simulink model "smd_openloop"  (R2026a)
settings: Solver=VariableStepAuto  StopTime=20
undefined symbols (not defined in the file): c, k, m
settings Model: Creator=tdxt  LastModifiedBy=tdxt

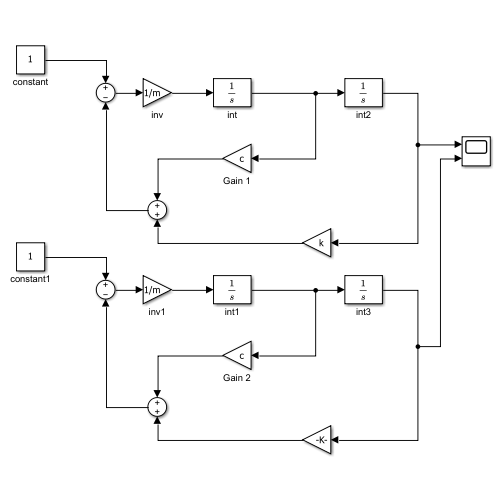
[thumbnail: Simulink's stored preview of the top-level diagram]
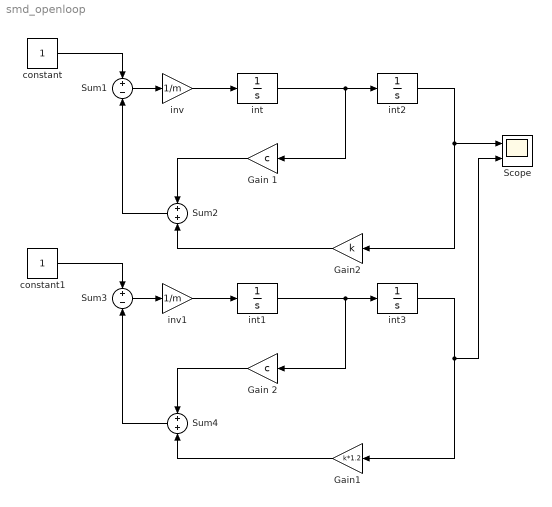
== system smd_openloop ==
  Gain 1 : Gain  Gain=c
  Gain 2 : Gain  Gain=c
  Gain1 : Gain  Gain=k*1.2
  Gain2 : Gain  Gain=k
  Scope : Scope  NumInputPorts=2
      settings: ActiveDisplayYMinimum=-0.14532946588879053  ActiveDisplayYMaximum=1.307965192999115
  Sum1 : Sum  Inputs=+-
  Sum2 : Sum
  Sum3 : Sum  Inputs=+-
  Sum4 : Sum
  constant : Constant
  constant1 : Constant
  int{,1..3} (4 alike) : Integrator
  inv : Gain  Gain=1/m
  inv1 : Gain  Gain=1/m
  wires:
  constant/1 -> Sum1/1
  int2/1 -> Gain2/1, Scope/1
  Gain2/1 -> Sum2/2
  Gain 1/1 -> Sum2/1
  Sum2/1 -> Sum1/2
  Sum1/1 -> inv/1
  inv/1 -> int/1
  int/1 -> int2/1, Gain 1/1
  int1/1 -> Gain 2/1, int3/1
  inv1/1 -> int1/1
  Sum3/1 -> inv1/1
  Sum4/1 -> Sum3/2
  Gain 2/1 -> Sum4/1
  Gain1/1 -> Sum4/2
  int3/1 -> Scope/2, Gain1/1
  constant1/1 -> Sum3/1
